simulink model "FUZZY_full_neurospora_model_leloup"  (R2015a)
settings: Solver=ode4  StartTime=0.0  StopTime=72  FixedStep=0.01  RelTol=1e-3
values from neighbouring files (symbols this model uses):
  k_1 = 0.5    [ALL_neurospora_init.m]    (also in FUZZY_deg_neurospora_init.m; FUZZY_tsc_neurospora_init.m; FUZZY_tsc_tsl_neurospora_init.m; FUZZY_tsl_neurospora_init.m)
  k_2 = 0.6    [ALL_neurospora_init.m]    (also in FUZZY_deg_neurospora_init.m; FUZZY_tsc_neurospora_init.m; FUZZY_tsc_tsl_neurospora_init.m; FUZZY_tsl_neurospora_init.m)
libraries: fuzblock x4
settings Model: Creator=jureb  LastModifiedBy=jureb

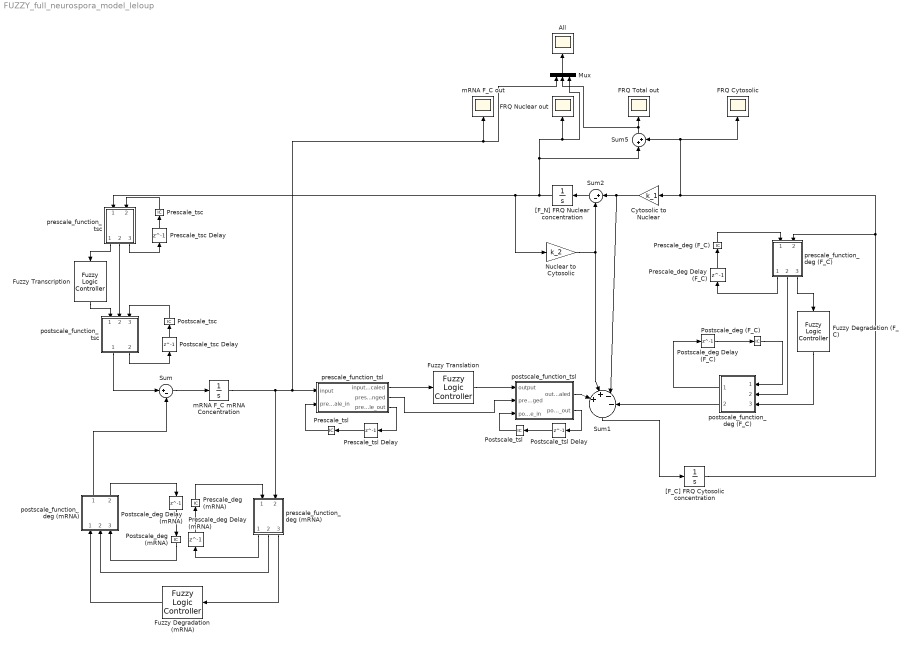
== system FUZZY_full_neurospora_model_leloup ==
  All : Scope
      settings: TimeRange=71.999776  YMin=0.5  YMax=8  SaveName=All
  Cytosolic to Nuclear : Gain  Gain=k_1
  FRQ Cytosolic : Scope
      settings: TimeRange=71.999776  YMin=0.5  YMax=10  SaveName=F_C2
  FRQ Nuclear out : Scope
      settings: TimeRange=71.999776  YMin=0  YMax=4.5  SaveName=F_N
  FRQ Total out : Scope
      settings: TimeRange=71.999776  YMin=0.5  YMax=10  SaveName=F_FL_full
  Fuzzy Degradation (F_C) : fuzblock/Fuzzy Logic  Controller  fis=deg
  Fuzzy Translation : fuzblock/Fuzzy Logic  Controller  fis=tsl
  Fuzzy Degradation (mRNA) : fuzblock/Fuzzy Logic  Controller  fis=deg
  Fuzzy Transcription : fuzblock/Fuzzy Logic  Controller  fis=tsc
  Mux : Mux  Inputs=3
  Nuclear to Cytosolic : Gain  Gain=k_2
  Postscale_deg (F_C) : InitialCondition  Value=2
  Postscale_deg (mRNA) : InitialCondition  Value=0.5
  Postscale_deg Delay (F_C) : Delay  DelayLength=1  InitialCondition=1
  Postscale_deg Delay (mRNA) : Delay  DelayLength=1  InitialCondition=1
  Postscale_tsc : InitialCondition  Value=1.3
  Postscale_tsc Delay : Delay  DelayLength=1  InitialCondition=1
  Postscale_tsl : InitialCondition  Value=2
  Postscale_tsl Delay : Delay  DelayLength=1  InitialCondition=1
  Prescale_deg (F_C) : InitialCondition  Value=4
  Prescale_deg (mRNA) : InitialCondition  Value=4
  Prescale_deg Delay (F_C) : Delay  DelayLength=1  InitialCondition=1  UseCircularBuffer=on
  Prescale_deg Delay (mRNA) : Delay  DelayLength=1  InitialCondition=1  UseCircularBuffer=on
  Prescale_tsc : InitialCondition  Value=5
  Prescale_tsc Delay : Delay  DelayLength=1  InitialCondition=1  UseCircularBuffer=on
  Prescale_tsl : InitialCondition  Value=5
  Prescale_tsl Delay : Delay  DelayLength=1  InitialCondition=1  UseCircularBuffer=on
  Sum : Sum  Inputs=|+-
  Sum1 : Sum  Inputs=|+|+|-|-
  Sum2 : Sum  Inputs=|+-
  Sum5 : Sum  Inputs=|++
  "[F_C] FRQ Cytosolic concentration " : Integrator  InitialCondition=1
  "[F_N] FRQ Nuclear concentration" : Integrator  InitialCondition=1
  mRNA F_C mRNA Concentration : Integrator  InitialCondition=1  LowerSaturationLimit=0
  mRNA F_C out : Scope
      settings: TimeRange=71.999776  YMin=0  YMax=6  SaveName=mRNA
  postscale_function_deg (F_C) : MATLAB Function  TreatAsAtomicUnit=on
  postscale_function_deg (mRNA) : MATLAB Function  TreatAsAtomicUnit=on
  postscale_function_tsc : MATLAB Function  TreatAsAtomicUnit=on
  postscale_function_tsl : MATLAB Function  TreatAsAtomicUnit=on
  prescale_function_deg (F_C) : MATLAB Function  TreatAsAtomicUnit=on
  prescale_function_deg (mRNA) : MATLAB Function  TreatAsAtomicUnit=on
  prescale_function_tsc : MATLAB Function  TreatAsAtomicUnit=on
  prescale_function_tsl : MATLAB Function  TreatAsAtomicUnit=on
  wires:
  postscale_function_tsc/1(output_postscaled) -> Sum/1
  Sum/1 -> mRNA F_C mRNA Concentration/1
  "[F_N] FRQ Nuclear concentration"/1 -> Nuclear to Cytosolic/1, prescale_function_tsc/1(input), Mux/3, FRQ Nuclear out/1, Sum5/1
  Sum1/1 -> "[F_C] FRQ Cytosolic concentration "/1
  Cytosolic to Nuclear/1 -> Sum1/3, Sum2/1
  Sum2/1 -> "[F_N] FRQ Nuclear concentration"/1
  Nuclear to Cytosolic/1 -> Sum1/2, Sum2/2
  Mux/1 -> All/1
  Sum5/1 -> Mux/2, FRQ Total out/1
  Postscale_deg (mRNA)/1 -> postscale_function_deg (mRNA)/3(postscale_in)
  postscale_function_deg (mRNA)/2(postscale_out) -> Postscale_deg Delay (mRNA)/1
  Postscale_deg Delay (mRNA)/1 -> Postscale_deg (mRNA)/1
  Fuzzy Degradation (mRNA)/1 -> postscale_function_deg (mRNA)/1(output)
  prescale_function_deg (mRNA)/1(prescale_out) -> Prescale_deg Delay (mRNA)/1
  Prescale_deg (mRNA)/1 -> prescale_function_deg (mRNA)/1(prescale_in)
  Prescale_deg Delay (mRNA)/1 -> Prescale_deg (mRNA)/1
  prescale_function_deg (mRNA)/3(input_prescaled) -> Fuzzy Degradation (mRNA)/1
  prescale_function_deg (mRNA)/2(prescale_changed) -> postscale_function_deg (mRNA)/2(prescale_changed)
  postscale_function_deg (mRNA)/1(output_postscaled) -> Sum/2
  "[F_C] FRQ Cytosolic concentration "/1 -> prescale_function_deg (F_C)/2(input), Sum5/2, FRQ Cytosolic/1, Cytosolic to Nuclear/1
  Postscale_deg (F_C)/1 -> postscale_function_deg (F_C)/1(postscale_in)
  postscale_function_deg (F_C)/1(postscale_out) -> Postscale_deg Delay (F_C)/1
  Postscale_deg Delay (F_C)/1 -> Postscale_deg (F_C)/1
  Fuzzy Degradation (F_C)/1 -> postscale_function_deg (F_C)/3(output)
  postscale_function_deg (F_C)/2(output_postscaled) -> Sum1/4
  prescale_function_deg (F_C)/1(prescale_out) -> Prescale_deg Delay (F_C)/1
  Prescale_deg (F_C)/1 -> prescale_function_deg (F_C)/1(prescale_in)
  Prescale_deg Delay (F_C)/1 -> Prescale_deg (F_C)/1
  prescale_function_deg (F_C)/3(input_prescaled) -> Fuzzy Degradation (F_C)/1
  prescale_function_deg (F_C)/2(prescale_changed) -> postscale_function_deg (F_C)/2(prescale_changed)
  prescale_function_tsl/1(input_prescaled) -> Fuzzy Translation/1
  Prescale_tsl/1 -> prescale_function_tsl/2(prescale_in)
  prescale_function_tsl/3(prescale_out) -> Prescale_tsl Delay/1
  Prescale_tsl Delay/1 -> Prescale_tsl/1
  Postscale_tsl/1 -> postscale_function_tsl/3(postscale_in)
  postscale_function_tsl/2(postscale_out) -> Postscale_tsl Delay/1
  Postscale_tsl Delay/1 -> Postscale_tsl/1
  Fuzzy Translation/1 -> postscale_function_tsl/1(output)
  postscale_function_tsl/1(output_postscaled) -> Sum1/1
  prescale_function_tsl/2(prescale_changed) -> postscale_function_tsl/2(prescale_changed)
  mRNA F_C mRNA Concentration/1 -> prescale_function_deg (mRNA)/2(input), prescale_function_tsl/1(input), Mux/1, mRNA F_C out/1
  prescale_function_tsc/3(prescale_out) -> Prescale_tsc Delay/1
  Prescale_tsc/1 -> prescale_function_tsc/2(prescale_in)
  Postscale_tsc/1 -> postscale_function_tsc/3(postscale_in)
  postscale_function_tsc/2(postscale_out) -> Postscale_tsc Delay/1
  Prescale_tsc Delay/1 -> Prescale_tsc/1
  Postscale_tsc Delay/1 -> Postscale_tsc/1
  prescale_function_tsc/1(input_prescaled) -> Fuzzy Transcription/1
  Fuzzy Transcription/1 -> postscale_function_tsc/1(output)
  prescale_function_tsc/2(prescale_changed) -> postscale_function_tsc/2(prescale_changed)

== matlab function FUZZY_full_neurospora_model_leloup/postscale_function_tsc ==
  data: output input; prescale_changed input; output_postscaled output; postscale_in input; postscale_out output
function [output_postscaled, postscale_out] = postscale(output, prescale_changed, postscale_in)

postscale_out = postscale_in;
multiplier = 1.01;

if (prescale_changed == 1)
    postscale_out = postscale_out*multiplier;
end

output_postscaled = output*postscale_out;

== matlab function FUZZY_full_neurospora_model_leloup/postscale_function_deg (mRNA) ==
  data: output input; prescale_changed input; output_postscaled output; postscale_in input; postscale_out output
function [output_postscaled, postscale_out] = postscale(output,prescale_changed, postscale_in)

postscale_out = postscale_in;
multiplier = 1.01;

if (prescale_changed == 1)
    postscale_out = postscale_out*multiplier;
end

output_postscaled = output*postscale_out;

== matlab function FUZZY_full_neurospora_model_leloup/postscale_function_deg (F_C) ==
  data: postscale_in input; prescale_changed input; postscale_out output; output input; output_postscaled output
function [postscale_out, output_postscaled] = postscale(postscale_in,prescale_changed, output)

postscale_out = postscale_in;
multiplier = 1.01;

if (prescale_changed == 1)
    postscale_out = postscale_out*multiplier;
end

output_postscaled = output*postscale_out;

== matlab function FUZZY_full_neurospora_model_leloup/prescale_function_deg (mRNA) ==
  data: prescale_in input; prescale_out output; prescale_changed output; input input; input_prescaled output
function [prescale_out, prescale_changed, input_prescaled] = prescale(prescale_in, input)

prescale_out = prescale_in;
multiplier = 1.01;
prescale_changed = 0;

if (input >= 0.9*prescale_in)
    prescale_out = prescale_in*multiplier;
    prescale_changed = 1;
end

input_prescaled = input/prescale_out;

== matlab function FUZZY_full_neurospora_model_leloup/prescale_function_deg (F_C) ==
  data: prescale_in input; prescale_out output; prescale_changed output; input input; input_prescaled output
function [prescale_out, prescale_changed, input_prescaled] = prescale(prescale_in, input)

prescale_out = prescale_in;
multiplier = 1.01;
prescale_changed = 0;

if (input >= 0.9*prescale_in)
    prescale_out = prescale_in*multiplier;
    prescale_changed = 1;
end

input_prescaled = input/prescale_out;

== matlab function FUZZY_full_neurospora_model_leloup/postscale_function_tsl ==
  data: output input; prescale_changed input; output_postscaled output; postscale_in input; postscale_out output
function [output_postscaled, postscale_out] = postscale(output, prescale_changed, postscale_in)

postscale_out = postscale_in;
multiplier = 1.01;

if (prescale_changed == 1)
    postscale_out = postscale_out*multiplier;
end

output_postscaled = output*postscale_out;

== matlab function FUZZY_full_neurospora_model_leloup/prescale_function_tsl ==
  data: input input; input_prescaled output; prescale_changed output; prescale_in input; prescale_out output
function [input_prescaled, prescale_changed, prescale_out] = prescale(input, prescale_in)

prescale_out = prescale_in;
multiplier = 1.01;
prescale_changed = 0;

if (input >= 0.9*prescale_in)
    prescale_out = prescale_in*multiplier;
    prescale_changed = 1;
end
    
input_prescaled = input/prescale_out;

== matlab function FUZZY_full_neurospora_model_leloup/prescale_function_tsc ==
  data: input input; input_prescaled output; prescale_changed output; prescale_in input; prescale_out output
function [input_prescaled, prescale_changed, prescale_out] = prescale(input, prescale_in)

prescale_out = prescale_in;
multiplier = 1.01;
prescale_changed = 0;

if (input >= 0.9*prescale_in)
    prescale_out = prescale_in*multiplier;
    prescale_changed = 1;
end

input_prescaled = input/prescale_out;
